simulink model "pattern_follow_body_frame"  (R2017a)
settings: Solver=FixedStepAuto  StartTime=0.0  StopTime=100  FixedStep=0.01  RelTol=1e-3
undefined symbols (not defined in the file): CoordinateFrame, TypeMask, Velocity
libraries: robotlib x3, simulink x3
settings Model: Creator=bshang2  LastModifiedBy=bshang2

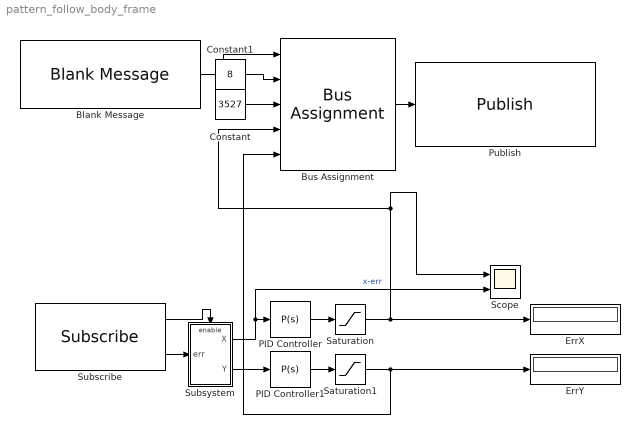
== system pattern_follow_body_frame ==
  Blank Message : robotlib/Blank Message  SourceLibraryInfo=This block requires Robotics System Toolbox  messageType=mavros_msgs/PositionTarget  SampleTime=inf
      settings: SourceProductBaseCode=RO
  Bus Assignment : BusAssignment  AssignedSignals=CoordinateFrame,TypeMask,Velocity.X,Velocity.Y
  Constant : Constant  Value=3527  OutDataTypeStr=uint16
  Constant1 : Constant  Value=8  OutDataTypeStr=uint8
  ErrX : Display
  ErrY : Display
  PID Controller : simulink/Continuous/PID Controller  Controller=P  TimeDomain=Continuous-time  SampleTime=-1  IntegratorMethod=Forward Euler  FilterMethod=Forward Euler  Form=Parallel  UseFilter=on  ControllerParametersSource=internal  P=-0.01  I=1  D=0  N=100  InitialConditionSource=internal  InitialConditionForIntegrator=0  InitialConditionForFilter=0  ExternalReset=none  LimitOutput=off  UpperSaturationLimit=inf  LowerSaturationLimit=-inf  LinearizeAsGain=on  AntiWindupMode=none  Kb=1  TrackingMode=off  Kt=1  PParamMin=[]  PParamMax=[]  IParamMin=[]  IParamMax=[]  DParamMin=[]  DParamMax=[]  NParamMin=[]  NParamMax=[]  KbParamMin=[]  KbParamMax=[]  KtParamMin=[]  KtParamMax=[]  POutMin=[]  POutMax=[]  IOutMin=[]  IOutMax=[]  DOutMin=[]  DOutMax=[]  NOutMin=[]  NOutMax=[]  KbOutMin=[]  KbOutMax=[]  KtOutMin=[]  KtOutMax=[]  IntegratorOutMin=[]  IntegratorOutMax=[]  FilterOutMin=[]  FilterOutMax=[]  SumOutMin=[]  SumOutMax=[]  SumI1OutMin=[]  SumI1OutMax=[]  SumI2OutMin=[]  SumI2OutMax=[]  SumI3OutMin=[]  SumI3OutMax=[]  SumDOutMin=[]  SumDOutMax=[]  SaturationOutMin=[]  SaturationOutMax=[]  IntegratorContinuousStateAttributes=''  IntegratorStateMustResolveToSignalObject=off  IntegratorRTWStateStorageClass=Auto  FilterContinuousStateAttributes=''  FilterStateMustResolveToSignalObject=off  FilterRTWStateStorageClass=Auto  DifferentiatorICPrevScaledInput=0  DifferentiatorOutMin=[]  DifferentiatorOutMax=[]  InitialConditionSetting=State (most efficient)
  PID Controller1 : simulink/Continuous/PID Controller  Controller=P  TimeDomain=Continuous-time  SampleTime=-1  IntegratorMethod=Forward Euler  FilterMethod=Forward Euler  Form=Parallel  UseFilter=on  ControllerParametersSource=internal  P=0.01  I=1  D=0  N=100  InitialConditionSource=internal  InitialConditionForIntegrator=0  InitialConditionForFilter=0  ExternalReset=none  LimitOutput=off  UpperSaturationLimit=inf  LowerSaturationLimit=-inf  LinearizeAsGain=on  AntiWindupMode=none  Kb=1  TrackingMode=off  Kt=1  PParamMin=[]  PParamMax=[]  IParamMin=[]  IParamMax=[]  DParamMin=[]  DParamMax=[]  NParamMin=[]  NParamMax=[]  KbParamMin=[]  KbParamMax=[]  KtParamMin=[]  KtParamMax=[]  POutMin=[]  POutMax=[]  IOutMin=[]  IOutMax=[]  DOutMin=[]  DOutMax=[]  NOutMin=[]  NOutMax=[]  KbOutMin=[]  KbOutMax=[]  KtOutMin=[]  KtOutMax=[]  IntegratorOutMin=[]  IntegratorOutMax=[]  FilterOutMin=[]  FilterOutMax=[]  SumOutMin=[]  SumOutMax=[]  SumI1OutMin=[]  SumI1OutMax=[]  SumI2OutMin=[]  SumI2OutMax=[]  SumI3OutMin=[]  SumI3OutMax=[]  SumDOutMin=[]  SumDOutMax=[]  SaturationOutMin=[]  SaturationOutMax=[]  IntegratorContinuousStateAttributes=''  IntegratorStateMustResolveToSignalObject=off  IntegratorRTWStateStorageClass=Auto  FilterContinuousStateAttributes=''  FilterStateMustResolveToSignalObject=off  FilterRTWStateStorageClass=Auto  DifferentiatorICPrevScaledInput=0  DifferentiatorOutMin=[]  DifferentiatorOutMax=[]  InitialConditionSetting=State (most efficient)
  Publish : robotlib/Publish  SourceLibraryInfo=This block requires Robotics System Toolbox  topicSource=Select from ROS network  topic=/mavros/setpoint_raw/local  messageType=mavros_msgs/PositionTarget  messageQueueLength=1
      settings: SourceProductBaseCode=RO
  Saturation : Saturate  UpperLimit=0.3  LowerLimit=-0.3
  Saturation1 : Saturate  UpperLimit=0.3  LowerLimit=-0.3
  Scope : Scope  NumInputPorts=2
  Subscribe : robotlib/Subscribe  SourceLibraryInfo=This block requires Robotics System Toolbox  topicSource=Select from ROS network  topic=/matlab/err  messageType=geometry_msgs/Pose2D  sampleTime=-1  messageQueueLength=1
      settings: SourceProductBaseCode=RO
  Subsystem : Subsystem
  wires:
  Blank Message/1 -> Bus Assignment/1
  Saturation/1 -> ErrX/1, Bus Assignment/4, Scope/1
  Bus Assignment/1 -> Publish/1
  Subscribe/2 -> Subsystem/1(err)
  Subsystem/1(X) -> Scope/2, PID Controller/1  "x-err"
  Subsystem/2(Y) -> PID Controller1/1
  Subscribe/1 -> Subsystem/Enable
  PID Controller/1 -> Saturation/1
  PID Controller1/1 -> Saturation1/1
  Saturation1/1 -> Bus Assignment/5, ErrY/1
  Constant/1 -> Bus Assignment/3
  Constant1/1 -> Bus Assignment/2

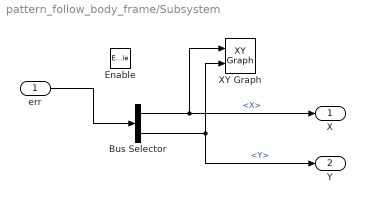
== system pattern_follow_body_frame/Subsystem ==
  err : Inport
  Enable : EnablePort
  Bus Selector : BusSelector  OutputSignals=X,Y
  XY Graph : simulink/Sinks/XY Graph  xmin=-100  xmax=100  ymin=-100  ymax=100  st=-1
  X : Outport
  Y : Outport  Port=2
  wires:
  err/1 -> Bus Selector/1
  Bus Selector/1 -> X/1, XY Graph/1  "<X>"
  Bus Selector/2 -> Y/1, XY Graph/2  "<Y>"
